simulink model "linear_control"  (R2021a)
settings: Solver=ode3  StartTime=0.0  StopTime=50  FixedStep=0.005  RelTol=1e-3
values from neighbouring files (symbols this model uses):
  a1 = 0.2634    [inital_for_newsimu.m]
  a2 = 1.6279    [inital_for_newsimu.m]
  a3 = 25.6488    [inital_for_newsimu.m]
  b1 = 0.531    [inital_for_newsimu.m]
  b2 = 5.3292    [inital_for_newsimu.m]
  b3 = 0.531    [inital_for_newsimu.m]
  b4 = 0.1157    [inital_for_newsimu.m]
  ce = 0.3010    (= 0.301)    [inital_for_newsimu.m]
  cp = 0.4804    [inital_for_newsimu.m]
  ct = 0.3410    (= 0.341)    [inital_for_newsimu.m]
  epsilon_d = epsilon    (= 0)    [inital_for_newsimu.m]
  K = [12.9295296815  7.11560022293  -3.04875118463e-16  -1.33966963984e-16; -1.57177988065e-15  -1.34451364306e-15  15.7580658816  2.56621295813]    [data0817三通道升降正弦偏航匀速实验.mat]
  K_psi2theta = [1.8 0.2]    [data0817三通道升降正弦偏航匀速实验.mat]    (also in inital_for_newsimu.m = [1.8,0.2])
libraries: dspsrcs4 x6, simulink x1
settings Model: SimulationMode=external  ExtModeTrigDuration=200000  Creator=5420  LastModifiedBy=DELL
settings SolverCC: AlgebraicLoopSolver=TrustRegion
settings DataIOCC: LimitDataPoints=on  SaveFormat=Array  SignalLoggingSaveFormat=ModelDataLogs  ReturnWorkspaceOutputs=off  SignalLoggingName=sigsOut
settings OptimizationCC: ExpressionDepthLimit=2147483647  InitFltsAndDblsToZero=on
settings DebuggingCC: SaveWithParameterizedLinksMsg=none  UnderspecifiedInitializationDetection=Classic  MergeDetectMultiDrivingBlocksExec=none  SignalResolutionControl=TryResolveAllWithWarning  MultiTaskDSMMsg=warning  MultiTaskCondExecSysMsg=none  StateNameClashWarn=warning  SFUnexpectedBacktrackingDiag=warning  SFNoUnconditionalDefaultTransitionDiag=warning  SFExecutionAtInitializationDiag=none  SFMachineParentedDataDiag=warning  ArithmeticOperatorsInVariantConditions=warning
settings ModelReferenceCC: PropagateSignalLabelsOutOfModel=off
settings SFSimCC: SimUseLocalCustomCode=off  CustomCodeUndefinedFunction=UseInterfaceOnly
settings RTWCC: Description=Simulink Desktop Real-Time  SystemTargetFile=sldrt.tlc  TemplateMakefile=sldrt.tmf  RTWUseLocalCustomCode=off  RTWCompilerOptimization=on
settings CodeAppCC: MaxIdLength=95  StateflowObjectComments=on
settings SimulinkDesktopRealTimeCC: TargetPreCompLibLocation=D:\Program Files (x86)\MatlabR21019b\toolbox\sldrt\lib\win64  TargetLangStandard=C89/C90 (ANSI)  ModelReferenceCompliant=off  CompOptLevelCompliant=off  SupportVariableSizeSignals=off
settings ConfigComp: CovMetricSettings=dw  CovSaveCumulativeToWorkspaceVar=on  CovSaveSingleToWorkspaceVar=on  CovExternalEMLEnable=off

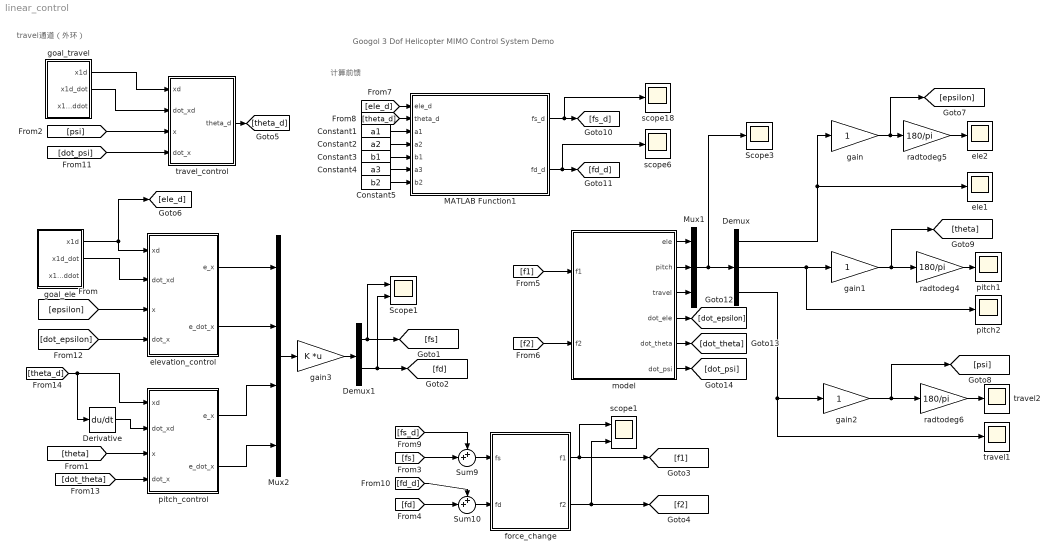
== system linear_control ==
  note: 计算前馈
  note: travel通道（外环）
  note: Googol 3 Dof Helicopter MIMO Control System Demo
  Constant1 : Constant  Value=a1
  Constant2 : Constant  Value=a2
  Constant3 : Constant  Value=b1
  Constant4 : Constant  Value=a3
  Constant5 : Constant  Value=b2
  Demux : Demux  Outputs=3
  Demux1 : Demux  Outputs=2
  Derivative : Derivative
  MATLAB Function1 : MATLAB Function  TreatAsAtomicUnit=on
  Mux1 : Mux  Inputs=3
  Mux2 : Mux
  Scope1 : Scope  NumInputPorts=2
  Scope3 : Scope
  Sum10 : Sum  Inputs=++|
  Sum9 : Sum  Inputs=++|
  ele1 : Scope
  ele2 : Scope
  elevation_control : Subsystem
  force_change : Subsystem
  gain : Gain
  gain1 : Gain
  gain2 : Gain
  gain3 : Gain  Gain=K  Multiplication=Matrix(K*u)
  goal_ele : Subsystem
  goal_travel : Subsystem
  model : Subsystem
  pitch1 : Scope
  pitch2 : Scope
  pitch_control : Subsystem
  radtodeg4 : Gain  Gain=180/pi
  radtodeg5 : Gain  Gain=180/pi
  radtodeg6 : Gain  Gain=180/pi
  scope1 : Scope  NumInputPorts=2
  scope18 : Scope
  scope6 : Scope
  travel1 : Scope
  travel2 : Scope
  travel_control : Subsystem
  wires:
  radtodeg5/1 -> ele2/1
  Demux/2 -> gain1/1, pitch2/1
  radtodeg6/1 -> travel2/1
  Demux/3 -> travel1/1, gain2/1
  Mux1/1 -> Scope3/1, Demux/1
  model/1("ele ") -> Mux1/1
  model/2(pitch) -> Mux1/2
  model/3(travel) -> Mux1/3
  Demux/1 -> gain/1, ele1/1
  radtodeg4/1 -> pitch1/1
  Mux2/1 -> gain3/1
  gain3/1 -> Demux1/1
  Demux1/1 -> Scope1/1, [fs]
  Demux1/2 -> Scope1/2, [fd]
  [f1] -> model/1(f1)
  [f2] -> model/2(f2)
  gain1/1 -> [theta], radtodeg4/1
  gain/1 -> [epsilon], radtodeg5/1
  gain2/1 -> radtodeg6/1, [psi]
  [theta_d] -> pitch_control/1(xd), Derivative/1
  [fs] -> Sum9/2
  [fd] -> Sum10/2
  [ele_d] -> MATLAB Function1/1(ele_d)
  [theta_d] -> MATLAB Function1/2(theta_d)
  Constant1/1 -> MATLAB Function1/3(a1)
  Constant2/1 -> MATLAB Function1/4(a2)
  Constant3/1 -> MATLAB Function1/5(b1)
  Constant4/1 -> MATLAB Function1/6(a3)
  Constant5/1 -> MATLAB Function1/7(b2)
  MATLAB Function1/1(fs_d) -> scope18/1, [fs_d]
  MATLAB Function1/2(fd_d) -> scope6/1, [fd_d]
  goal_travel/1(x1d) -> travel_control/1(xd)
  goal_travel/2(x1d_dot) -> travel_control/2(dot_xd)
  [psi] -> travel_control/3(x)
  goal_ele/1(x1d) -> [ele_d], elevation_control/1(xd)
  goal_ele/2(x1d_dot) -> elevation_control/2(dot_xd)
  [epsilon] -> elevation_control/3(x)
  Derivative/1 -> pitch_control/2(dot_xd)
  [theta] -> pitch_control/3(x)
  model/4("dot_ele ") -> [dot_epsilon]
  model/5(dot_theta) -> [dot_theta]
  model/6(dot_psi) -> [dot_psi]
  [dot_psi] -> travel_control/4(dot_x)
  [dot_theta] -> pitch_control/4(dot_x)
  [dot_epsilon] -> elevation_control/4(dot_x)
  [fs_d] -> Sum9/1
  [fd_d] -> Sum10/1
  elevation_control/1(e_x) -> Mux2/1
  elevation_control/2(e_dot_x) -> Mux2/2
  pitch_control/1(e_x) -> Mux2/3
  pitch_control/2(e_dot_x) -> Mux2/4
  travel_control/1(theta_d) -> [theta_d]
  force_change/1(f1) -> scope1/1, [f1]
  force_change/2(f2) -> scope1/2, [f2]
  Sum9/1 -> force_change/1(fs)
  Sum10/1 -> force_change/2(fd)

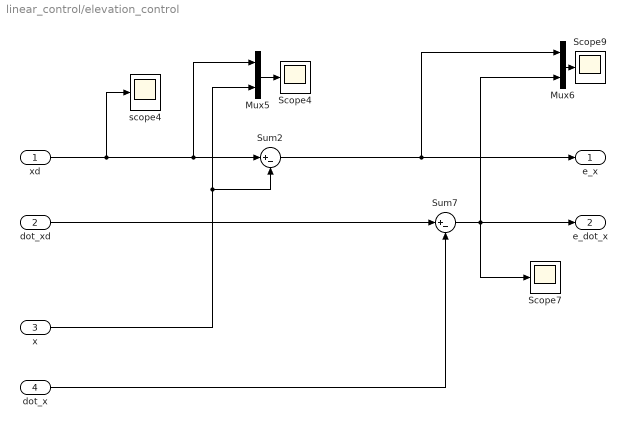
== system linear_control/elevation_control ==
  xd : Inport
  dot_xd : Inport  Port=2
  x : Inport  Port=3
  dot_x : Inport  Port=4
  Mux5 : Mux  Inputs=2
  Mux6 : Mux  Inputs=2
  Scope4 : Scope
  Scope7 : Scope
  Scope9 : Scope
  Sum2 : Sum  Inputs=|+-
  Sum7 : Sum  Inputs=|+-
  scope4 : Scope
  e_x : Outport
  e_dot_x : Outport  Port=2
  wires:
  xd/1 -> Mux5/1, Sum2/1, scope4/1
  Mux6/1 -> Scope9/1
  Mux5/1 -> Scope4/1
  dot_x/1 -> Sum7/2
  x/1 -> Mux5/2, Sum2/2
  Sum7/1 -> Mux6/2, e_dot_x/1, Scope7/1
  Sum2/1 -> e_x/1, Mux6/1
  dot_xd/1 -> Sum7/1

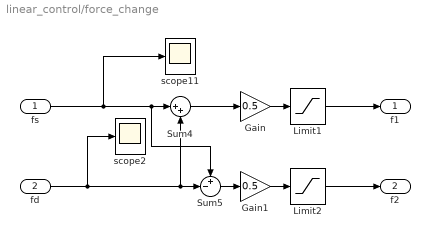
== system linear_control/force_change ==
  fs : Inport
  fd : Inport  Port=2
  Gain : Gain  Gain=0.5
  Gain1 : Gain  Gain=0.5
  Limit1 : Saturate  UpperLimit=4  LowerLimit=0.05
  Limit2 : Saturate  UpperLimit=4  LowerLimit=0.05
  Sum4 : Sum  Inputs=|++
  Sum5 : Sum  Inputs=+-|
  scope11 : Scope
  scope2 : Scope
  f1 : Outport
  f2 : Outport  Port=2
  wires:
  Gain1/1 -> Limit2/1
  fd/1 -> scope2/1, Sum5/2, Sum4/2
  fs/1 -> scope11/1, Sum5/1, Sum4/1
  Limit1/1 -> f1/1
  Sum5/1 -> Gain1/1
  Limit2/1 -> f2/1
  Gain/1 -> Limit1/1
  Sum4/1 -> Gain/1

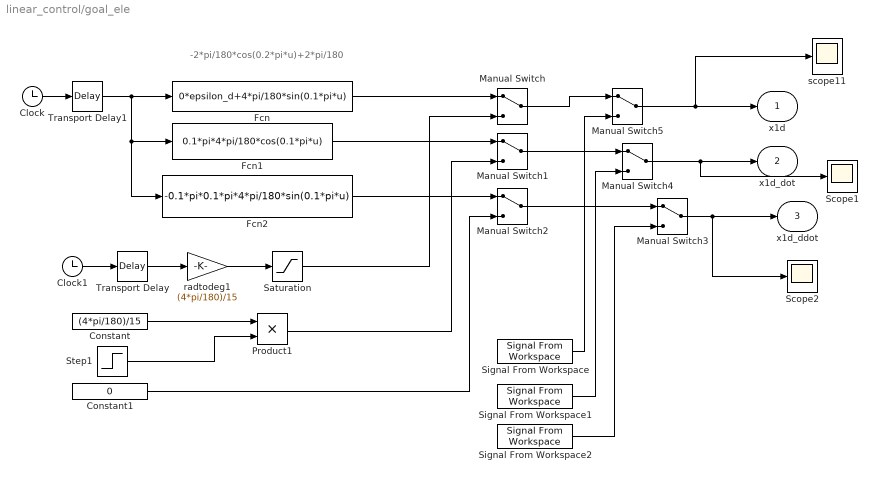
== system linear_control/goal_ele ==
  note: -2*pi/180*cos(0.2*pi*u)+2*pi/180
  Clock : Clock
  Clock1 : Clock
  Constant : Constant  Value=(4*pi/180)/15
  Constant1 : Constant  Value=0
  Fcn : Fcn  Expr=0*epsilon_d+4*pi/180*sin(0.1*pi*u)
  Fcn1 : Fcn  Expr=0.1*pi*4*pi/180*cos(0.1*pi*u)
  Fcn2 : Fcn  Expr=-0.1*pi*0.1*pi*4*pi/180*sin(0.1*pi*u)
  Manual Switch{,1..5} (6 alike) : ManualSwitch
  Product1 : Product  RndMeth=Zero
  Saturation : Saturate  UpperLimit=(4*pi/180)  LowerLimit=-(4*pi/180)
  Scope1 : Scope
  Scope2 : Scope
  Signal From Workspace : dspsrcs4/Signal From Workspace  X=epsilon  Ts=0.005  nsamps=1  OutputAfterFinalValue=Setting to zero  ignoreOrWarnInputAndFrameLengths=off  OutputFrames=on
  Signal From Workspace1 : dspsrcs4/Signal From Workspace  X=dot_epsilon  Ts=0.005  nsamps=1  OutputAfterFinalValue=Setting to zero  ignoreOrWarnInputAndFrameLengths=off  OutputFrames=on
  Signal From Workspace2 : dspsrcs4/Signal From Workspace  X=ddot_epsilon  Ts=0.005  nsamps=1  OutputAfterFinalValue=Setting to zero  ignoreOrWarnInputAndFrameLengths=off  OutputFrames=on
  Step1 : Step  Time=12  SampleTime=0
  Transport Delay : TransportDelay  DelayTime=12
  Transport Delay1 : TransportDelay  DelayTime=0
  radtodeg1 : Gain  Gain=(4*pi/180)/15
  scope11 : Scope
  x1d : Outport
  x1d_dot : Outport  Port=2
  x1d_ddot : Outport  Port=3
  wires:
  Clock/1 -> Transport Delay1/1
  Clock1/1 -> Transport Delay/1
  Transport Delay/1 -> radtodeg1/1
  radtodeg1/1 -> Saturation/1
  Fcn/1 -> Manual Switch/1
  Fcn1/1 -> Manual Switch1/1
  Fcn2/1 -> Manual Switch2/1
  Manual Switch2/1 -> Manual Switch3/1
  Saturation/1 -> Manual Switch/2
  Constant1/1 -> Manual Switch2/2
  Constant/1 -> Product1/1
  Step1/1 -> Product1/2
  Product1/1 -> Manual Switch1/2
  Transport Delay1/1 -> Fcn1/1, Fcn2/1, Fcn/1
  Signal From Workspace2/1 -> Manual Switch3/2
  Manual Switch3/1 -> Scope2/1, x1d_ddot/1
  Signal From Workspace1/1 -> Manual Switch4/2
  Manual Switch1/1 -> Manual Switch4/1
  Manual Switch4/1 -> Scope1/1, x1d_dot/1
  Manual Switch/1 -> Manual Switch5/1
  Signal From Workspace/1 -> Manual Switch5/2
  Manual Switch5/1 -> scope11/1, x1d/1

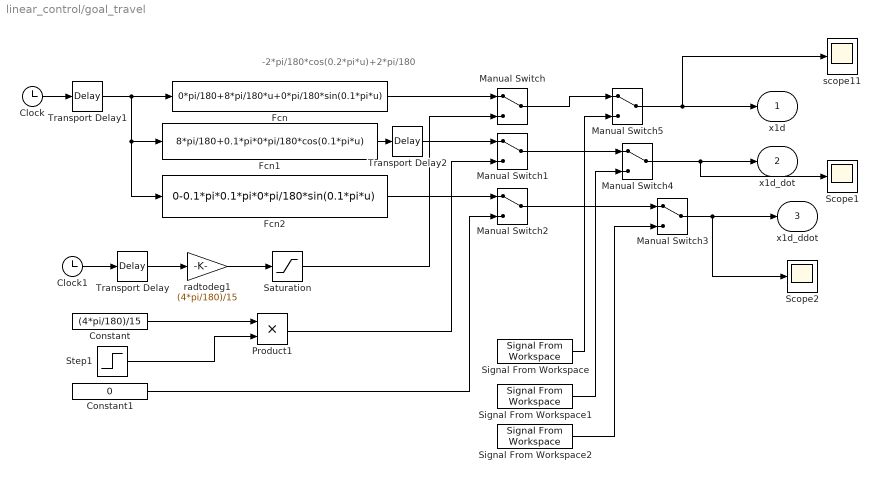
== system linear_control/goal_travel ==
  note: -2*pi/180*cos(0.2*pi*u)+2*pi/180
  Clock : Clock
  Clock1 : Clock
  Constant : Constant  Value=(4*pi/180)/15
  Constant1 : Constant  Value=0
  Fcn : Fcn  Expr=0*pi/180+8*pi/180*u+0*pi/180*sin(0.1*pi*u)
  Fcn1 : Fcn  Expr=8*pi/180+0.1*pi*0*pi/180*cos(0.1*pi*u)
  Fcn2 : Fcn  Expr=0-0.1*pi*0.1*pi*0*pi/180*sin(0.1*pi*u)
  Manual Switch{,1..5} (6 alike) : ManualSwitch
  Product1 : Product  RndMeth=Zero
  Saturation : Saturate  UpperLimit=(4*pi/180)  LowerLimit=-(4*pi/180)
  Scope1 : Scope
  Scope2 : Scope
  Signal From Workspace : dspsrcs4/Signal From Workspace  X=epsilon  Ts=0.005  nsamps=1  OutputAfterFinalValue=Setting to zero  ignoreOrWarnInputAndFrameLengths=off  OutputFrames=on
  Signal From Workspace1 : dspsrcs4/Signal From Workspace  X=dot_epsilon  Ts=0.005  nsamps=1  OutputAfterFinalValue=Setting to zero  ignoreOrWarnInputAndFrameLengths=off  OutputFrames=on
  Signal From Workspace2 : dspsrcs4/Signal From Workspace  X=ddot_epsilon  Ts=0.005  nsamps=1  OutputAfterFinalValue=Setting to zero  ignoreOrWarnInputAndFrameLengths=off  OutputFrames=on
  Step1 : Step  Time=12  SampleTime=0
  Transport Delay : TransportDelay  DelayTime=12
  Transport Delay1 : TransportDelay  DelayTime=0
  Transport Delay2 : TransportDelay  DelayTime=0
  radtodeg1 : Gain  Gain=(4*pi/180)/15
  scope11 : Scope
  x1d : Outport
  x1d_dot : Outport  Port=2
  x1d_ddot : Outport  Port=3
  wires:
  Clock/1 -> Transport Delay1/1
  Clock1/1 -> Transport Delay/1
  Transport Delay/1 -> radtodeg1/1
  radtodeg1/1 -> Saturation/1
  Manual Switch2/1 -> Manual Switch3/1
  Saturation/1 -> Manual Switch/2
  Constant1/1 -> Manual Switch2/2
  Constant/1 -> Product1/1
  Step1/1 -> Product1/2
  Product1/1 -> Manual Switch1/2
  Transport Delay1/1 -> Fcn1/1, Fcn2/1, Fcn/1
  Signal From Workspace2/1 -> Manual Switch3/2
  Manual Switch3/1 -> Scope2/1, x1d_ddot/1
  Signal From Workspace1/1 -> Manual Switch4/2
  Manual Switch1/1 -> Manual Switch4/1
  Manual Switch4/1 -> Scope1/1, x1d_dot/1
  Manual Switch/1 -> Manual Switch5/1
  Signal From Workspace/1 -> Manual Switch5/2
  Manual Switch5/1 -> scope11/1, x1d/1
  Fcn/1 -> Manual Switch/1
  Fcn1/1 -> Transport Delay2/1
  Fcn2/1 -> Manual Switch2/1
  Transport Delay2/1 -> Manual Switch1/1

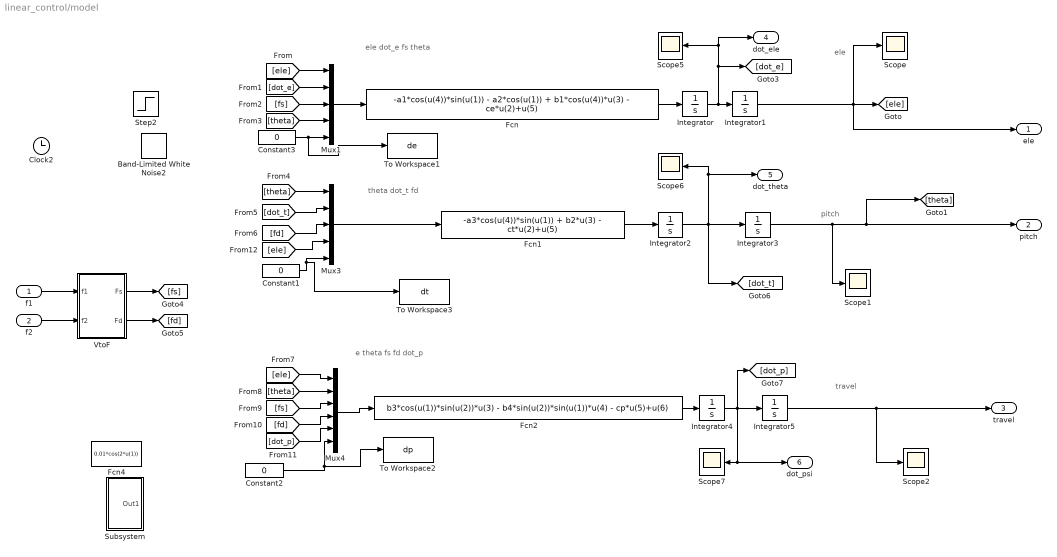
== system linear_control/model ==
  note: e
      | theta
      | fs
      | fd
      | dot_p
  note: ele
      | dot_e
      | fs
      | theta
  note: travel
  note: pitch
  note: ele
  note: theta
      | dot_t
      | fd
  f1 : Inport
  f2 : Inport  Port=2
  Band-Limited White Noise2 : simulink/Sources/Band-Limited White Noise  Cov=[0.001]  Ts=1  seed=[23341]
  Clock2 : Clock
      settings: Decimation=30
  Constant1 : Constant  Value=0
  Constant2 : Constant  Value=0
  Constant3 : Constant  Value=0
  Fcn : Fcn  Expr=-a1*cos(u(4))*sin(u(1)) - a2*cos(u(1)) + b1*cos(u(4))*u(3) - ce*u(2)+u(5)
  Fcn1 : Fcn  Expr=-a3*cos(u(4))*sin(u(1)) + b2*u(3) - ct*u(2)+u(5)
  Fcn2 : Fcn  Expr=b3*cos(u(1))*sin(u(2))*u(3) - b4*sin(u(2))*sin(u(1))*u(4) - cp*u(5)+u(6)
  Fcn4 : Fcn  Expr=0.01*cos(2*u(1))
  Integrator{,2..5} (5 alike) : Integrator
  Integrator1 : Integrator  InitialCondition=-0.545
  Mux1 : Mux  Inputs=5
  Mux3 : Mux  Inputs=5
  Mux4 : Mux  Inputs=6
  Scope{,1..2,5..7} (6 alike) : Scope
  Step2 : Step  Time=40  After=0.2  SampleTime=0
  Subsystem : Subsystem
  To Workspace1 : ToWorkspace  VariableName=de  SampleTime=-1
  To Workspace2 : ToWorkspace  VariableName=dp  SampleTime=-1
  To Workspace3 : ToWorkspace  VariableName=dt  SampleTime=-1
  VtoF : Subsystem
  "ele " : Outport  VectorParamsAs1DForOutWhenUnconnected=off
  pitch : Outport  Port=2  VectorParamsAs1DForOutWhenUnconnected=off
  travel : Outport  Port=3  VectorParamsAs1DForOutWhenUnconnected=off
  "dot_ele " : Outport  Port=4  VectorParamsAs1DForOutWhenUnconnected=off
  dot_theta : Outport  Port=5  VectorParamsAs1DForOutWhenUnconnected=off
  dot_psi : Outport  Port=6  VectorParamsAs1DForOutWhenUnconnected=off
  wires:
  Integrator1/1 -> "ele "/1, Scope/1, [ele]
  Fcn/1 -> Integrator/1
  Integrator3/1 -> pitch/1, [theta], Scope1/1
  Integrator/1 -> "dot_ele "/1, Scope5/1, [dot_e], Integrator1/1
  Fcn1/1 -> Integrator2/1
  Fcn2/1 -> Integrator4/1
  Integrator4/1 -> dot_psi/1, Scope7/1, [dot_p], Integrator5/1
  Mux1/1 -> Fcn/1
  Mux4/1 -> Fcn2/1
  [ele] -> Mux1/1
  [dot_e] -> Mux1/2
  VtoF/1(Fs) -> [fs]
  VtoF/2(Fd) -> [fd]
  [fs] -> Mux1/3
  [theta] -> Mux1/4
  [ele] -> Mux4/1
  [theta] -> Mux4/2
  [fs] -> Mux4/3
  [fd] -> Mux4/4
  [dot_p] -> Mux4/5
  Integrator2/1 -> dot_theta/1, Scope6/1, [dot_t], Integrator3/1
  f1/1 -> VtoF/1(f1)
  f2/1 -> VtoF/2(f2)
  Mux3/1 -> Fcn1/1
  [theta] -> Mux3/1
  [dot_t] -> Mux3/2
  [fd] -> Mux3/3
  [ele] -> Mux3/4
  Constant1/1 -> To Workspace3/1, Mux3/5
  Integrator5/1 -> travel/1, Scope2/1
  Constant3/1 -> To Workspace1/1, Mux1/5
  Constant2/1 -> To Workspace2/1, Mux4/6

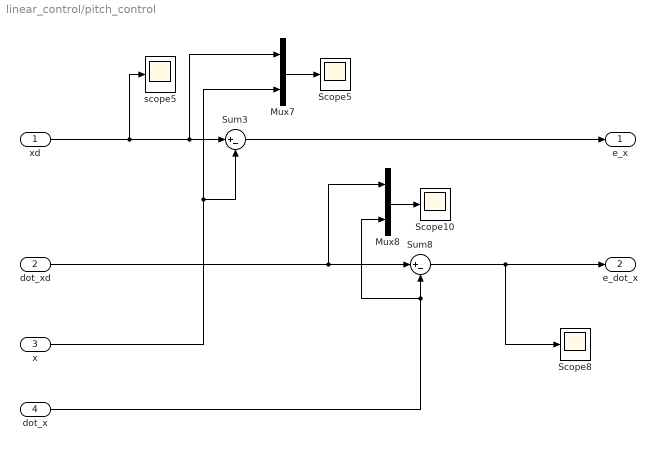
== system linear_control/pitch_control ==
  xd : Inport
  dot_xd : Inport  Port=2
  x : Inport  Port=3
  dot_x : Inport  Port=4
  Mux7 : Mux  Inputs=2
  Mux8 : Mux  Inputs=2
  Scope10 : Scope
  Scope5 : Scope
  Scope8 : Scope
  Sum3 : Sum  Inputs=|+-
  Sum8 : Sum  Inputs=|+-
  scope5 : Scope
  e_x : Outport
  e_dot_x : Outport  Port=2
  wires:
  Sum3/1 -> e_x/1
  dot_x/1 -> Sum8/2, Mux8/2
  Sum8/1 -> Scope8/1, e_dot_x/1
  xd/1 -> scope5/1, Mux7/1, Sum3/1
  x/1 -> Sum3/2, Mux7/2
  Mux8/1 -> Scope10/1
  dot_xd/1 -> Sum8/1, Mux8/1
  Mux7/1 -> Scope5/1

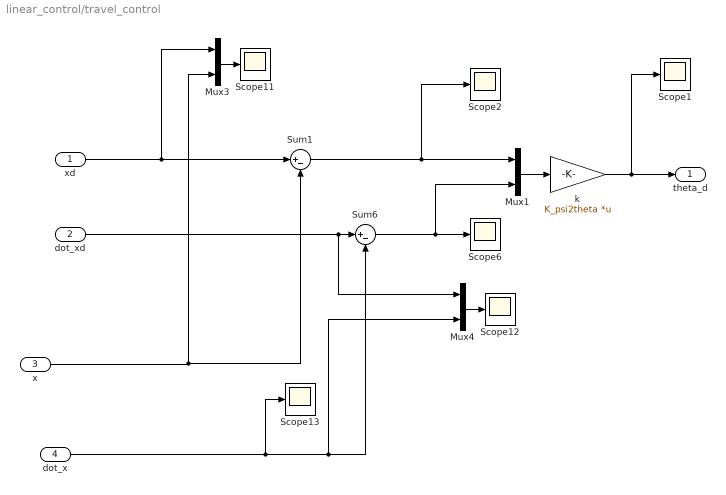
== system linear_control/travel_control ==
  xd : Inport
  dot_xd : Inport  Port=2
  x : Inport  Port=3
  dot_x : Inport  Port=4
  Mux1 : Mux  Inputs=2
  Mux3 : Mux  Inputs=2
  Mux4 : Mux  Inputs=2
  Scope{1..2,6,11..13} (6 alike) : Scope
  Sum1 : Sum  Inputs=|+-
  Sum6 : Sum  Inputs=|+-
  k : Gain  Gain=K_psi2theta  Multiplication=Matrix(K*u)
  theta_d : Outport
  wires:
  dot_xd/1 -> Mux4/1, Sum6/1
  x/1 -> Sum1/2, Mux3/2
  dot_x/1 -> Scope13/1, Mux4/2, Sum6/2
  Sum6/1 -> Mux1/2, Scope6/1
  Mux3/1 -> Scope11/1
  Mux4/1 -> Scope12/1
  Sum1/1 -> Mux1/1, Scope2/1
  xd/1 -> Mux3/1, Sum1/1
  Mux1/1 -> k/1
  k/1 -> Scope1/1, theta_d/1

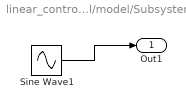
== system linear_control/model/Subsystem ==
  Sine Wave1 : Sin  Amplitude=0.01  SampleTime=0
  Out1 : Outport
  wires:
  Sine Wave1/1 -> Out1/1

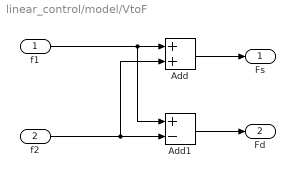
== system linear_control/model/VtoF ==
  f1 : Inport
  f2 : Inport  Port=2
  Add : Sum
  Add1 : Sum  Inputs=+-
  Fs : Outport  VectorParamsAs1DForOutWhenUnconnected=off
  Fd : Outport  Port=2  VectorParamsAs1DForOutWhenUnconnected=off
  wires:
  Add1/1 -> Fd/1
  f2/1 -> Add1/2, Add/2
  f1/1 -> Add1/1, Add/1
  Add/1 -> Fs/1

== matlab function linear_control/MATLAB Function1 ==
  data: fs_d output; ele_d input; fd_d output; theta_d input; a1 input; a2 input; b1 input; a3 input; b2 input
function [fs_d,fd_d] = fcn(ele_d,theta_d,a1,a2,b1,a3,b2)
theta = theta_d;
epsilon = ele_d;

fs_d = (a1*cos(theta)*sin(epsilon)+a2*cos(epsilon))/(b1*cos(theta));
fd_d = a3*cos(epsilon)*sin(theta)/b2;
